simulink model "Quadcopter"  (R2023b)
settings: Solver=VariableStepAuto  StartTime=0.0  StopTime=30  RelTol=1e-3
values from neighbouring files (symbols this model uses):
  Pobs1x = zeros(1, length(Ob1))    [UAVsAnimation.m]    (also in UAVs_TwoObstacles.m)
  Pobs1y = zeros(1, length(Ob1))    [UAVsAnimation.m]    (also in UAVs_TwoObstacles.m)
  Pobs1z = zeros(1, length(Ob1))    [UAVsAnimation.m]    (also in UAVs_TwoObstacles.m)
  Pobs2x = zeros(1, length(Ob2))    [UAVsAnimation.m]    (also in UAVs_TwoObstacles.m)
  Pobs2y = zeros(1, length(Ob2))    [UAVsAnimation.m]    (also in UAVs_TwoObstacles.m)
  Pobs2z = zeros(1, length(Ob2))    [UAVsAnimation.m]    (also in UAVs_TwoObstacles.m)
  X = x(:,1)    [UAVs_TwoObstacles.m]
  xd = cell2mat(Xd)    [UAVs_TwoObstacles.m]
  Y = x(:,2)    [UAVs_TwoObstacles.m]
  yd = cell2mat(Yd)    [UAVs_TwoObstacles.m]
  Z = x(:,3)    [UAVs_TwoObstacles.m]
  zd = cell2mat(Zd)    [UAVs_TwoObstacles.m]
libraries: sim3dlib x5, slpidlib x1
settings Model: Creator=The MathWorks, Inc.  LastModifiedBy=galil
settings OptimizationCC: ReuseModelBlockBuffer=off

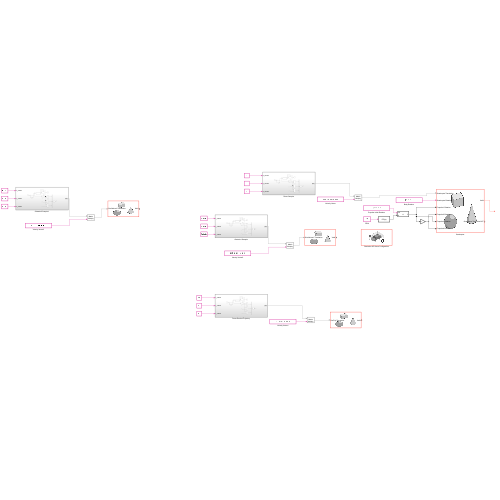
[thumbnail: Simulink's stored preview of the top-level diagram]
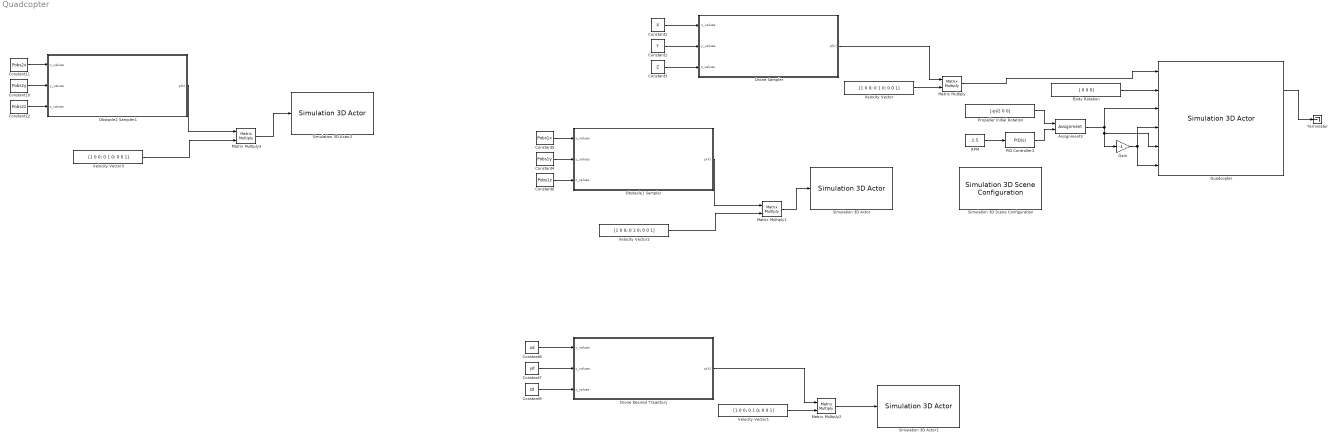
== system Quadcopter ==
  Assignment3 : Assignment  DiagnosticForDimensions=Warning  IndexOptions=Index vector (dialog)  Indices=3  OutputSizes=1
  Body Rotation : Constant  Value=[ 0 0 0]  VectorParams1D=off
  Constant1 : Constant  Value=Y
  Constant10 : Constant  Value=Pobs2y
  Constant11 : Constant  Value=Pobs2x
  Constant12 : Constant  Value=Pobs2z
  Constant2 : Constant  Value=X
  Constant3 : Constant  Value=Z
  Constant4 : Constant  Value=Pobs1y
  Constant5 : Constant  Value=Pobs1x
  Constant6 : Constant  Value=Pobs1z
  Constant7 : Constant  Value=yd
  Constant8 : Constant  Value=xd
  Constant9 : Constant  Value=zd
  Drone Desired Trajectory : Subsystem
  Drone Sampler : Subsystem
  Gain : Gain  Gain=-1
  Matrix Multiply{,1..3} (4 alike) : Product  Multiplication=Matrix(*)
  Obstacle1 Sampler : Subsystem
  Obstacle2 Sampler1 : Subsystem
  PID Controller3 : slpidlib/PID Controller  Controller=PID  Form=Parallel  TimeDomain=Continuous-time  UseExternalTs=off  SampleTime=-1  IntegratorMethod=Forward Euler  FilterMethod=Forward Euler  ControllerParametersSource=internal  P=0  I=1  UseKiTs=off  D=0  N=100  UseFilter=on  TunerSelectOption=Transfer Function Based (PID Tuner App)  InitialConditionSource=internal  InitialConditionForIntegrator=0  InitialConditionForFilter=0  DifferentiatorICPrevScaledInput=0  ExternalReset=none  TrackingMode=off  Kt=1  LimitOutput=off  SatLimitsSource=internal  UpperSaturationLimit=inf  LowerSaturationLimit=-inf  LinearizeAsGain=on  AntiWindupMode=none  Kb=1  LimitIntegrator=off  UpperIntegratorSaturationLimit=inf  LowerIntegratorSaturationLimit=-inf  POutMin=[]  POutMax=[]  IOutMin=[]  IOutMax=[]  DOutMin=[]  DOutMax=[]  NOutMin=[]  NOutMax=[]  SumOutMin=[]  SumOutMax=[]  SaturationOutMin=[]  SaturationOutMax=[]  PParamMin=[]  PParamMax=[]  IParamMin=[]  IParamMax=[]  DParamMin=[]  DParamMax=[]  NParamMin=[]  NParamMax=[]  KbParamMin=[]  KbParamMax=[]  KtParamMin=[]  KtParamMax=[]  KbOutMin=[]  KbOutMax=[]  KtOutMin=[]  KtOutMax=[]  IntegratorOutMin=[]  IntegratorOutMax=[]  FilterOutMin=[]  FilterOutMax=[]  SumI1OutMin=[]  SumI1OutMax=[]  SumI2OutMin=[]  SumI2OutMax=[]  SumI3OutMin=[]  SumI3OutMax=[]  SumI4OutMin=[]  SumI4OutMax=[]  SumDOutMin=[]  SumDOutMax=[]  DifferentiatorOutMin=[]  DifferentiatorOutMax=[]  FilterDiffOutCoefMin=[]  FilterDiffOutCoefMax=[]  ReciprocalOutMin=[]  ReciprocalOutMax=[]  SumDenOutMin=[]  SumDenOutMax=[]  SumNumOutMin=[]  SumNumOutMax=[]  DivideOutMin=[]  DivideOutMax=[]  UdiffTsProdOutMin=[]  UdiffTsProdOutMax=[]  NTsProdOutMin=[]  NTsProdOutMax=[]  UintegralTsProdOutMin=[]  UintegralTsProdOutMax=[]  UngainTsProdOutMin=[]  UngainTsProdOutMax=[]  ClampingZeroOutDataTypeStr=Inherit: Inherit via back propagation  ClampingZeroOutMin=[]  ClampingZeroOutMax=[]  FilterDenConstantOutDataTypeStr=Inherit: Inherit via back propagation  FilterDenConstantOutMin=[]  FilterDenConstantOutMax=[]  PCopyOutDataTypeStr=Inherit: Inherit via back propagation  PCopyOutMin=[]  PCopyOutMax=[]  NCopyOutDataTypeStr=Inherit: Inherit via back propagation  NCopyOutMin=[]  NCopyOutMax=[]  IntegratorContinuousStateAttributes=''  IntegratorStateMustResolveToSignalObject=off  IntegratorRTWStateStorageClass=Auto  FilterContinuousStateAttributes=''  FilterStateMustResolveToSignalObject=off  FilterRTWStateStorageClass=Auto  ParallelPVariant=InternalParameters  IdealPVariant=Disabled  IVariant=InternalParameters  DVariant=InternalParameters  IntegratorVariant=Continuous  SatVariant=Disabled  AWVariant=Passthrough  PCopyVariant=Disabled  TRVariant=Disabled  FdbkBlocksVariant=Forward  IdealPFdbkVariant=Disabled  SatFdbkVariant=Disabled  DerivativeFilterVariant=ContFilter  NVariant=InternalParameters  NCopyVariant=Disabled  FilterICVariant=InternalICsFilter  IntegratorICVariant=InternalICs  ExternalResetVariant=Disabled  TRSumVariant=Passthrough  SumFdbkVariant=Disabled  SumVariant=Sum_PID  TsampFilterVariant=InternalTs  TsampNgainVariant=Passthrough  TsampIntegralVariant=Disabled_SignalSpec  ExternalSaturationOutDataTypeStr=Inherit: Same as second input
  Propeller Initial Rotation : Constant  Value=[-pi/2 0 0]  VectorParams1D=off
  Quadcopter : sim3dlib/Simulation 3D Actor  ActorName=Quadcopter  ParentName=Scene Origin  Operation=Create at setup  InitScriptText=|  SampleTime=-1  Translation=single([-3.5 0 1.7])  Rotation=single([0 0 0])  Scale=single([1 1 1])  InputsText=|  OutputsText=Quadcopter.Translation  aMode=5  ActorTag=Quadcopter  ActorType=Sim3dActor  ID=C
      InitScriptText=|
      | fileName = "QuadCopter_Body.stl";
      | Body = sim3d.Actor('ActorName', 'Body', ...
      |     'Mobility', sim3d.utils.MobilityTypes.Movable, ...
      |     'ActorClassId', sim3d.utils.SemanticType.Vehicle);
      | World.add(Body, Actor);
      | Body.load(fileName, [1 1 1]/100);
      | Body.Rotation = [-pi/2 0 0 ];
      | Body.Color = [0, 0, 1];
      | Translation = [0.425 0.425 0.15;
      |     -0.425 0.425 0.15;
      |     0.425 -0.425 0.15;
      |     -0.425 -0.425 0.15];
      | propellerFileName = "QuadCopter_Propeller.stl";
      | for propellerIndex = 1:4
      | actorName = sprintf('Propeller%d', propellerIndex);
      | Propeller = sim3d.Actor('ActorName',actorName, ...
      |     'Mobility', sim3d.utils.MobilityTypes.Movable, ...
      |     'ActorClassId', sim3d.utils.SemanticType.Vehicle);
      | World.add(Propeller, Actor);
      | Propeller.load(propellerFileName, [1 1 1]/100);
      | Propeller.Color = [1, 0, 0];
      | Propeller.Translation = Translation(propellerIndex, :);
      | Propeller.Rotation = [-pi/2 0 0 ];
      | Actor.save("quadcopter.mat")
      | end
      InputsText=|
      | Quadcopter.Translation
      | Quadcopter.Rotation   
      | Propeller1.Rotation   
      | Propeller2.Rotation   
      | Propeller3.Rotation   
      | Propeller4.Rotation
      settings: LibrarySourceBlock=sl3dlib/Simulation 3D/Simulation 3D Actor
  RPM : Constant  Value=2.5
  Simulation 3D Actor : sim3dlib/Simulation 3D Actor  ActorName=Sim3dActor1  ParentName=Scene Origin  Operation=Create at setup  InitScriptText=|  SampleTime=-1  Translation=single([0 0 0])  Rotation=single([0 0 0])  Scale=single([1 1 1])  InputsText=Sim3dActor1.Translation  aMode=5  ActorTag=Sim3dActor1  ActorType=Sim3dActor  ID=1
      | Sim3dActor1 = sim3d.Actor('ActorName','Sim3dActor1', ...
      |     'Mobility', sim3d.utils.MobilityTypes.Movable, ...
      |     'ActorClassId', sim3d.utils.SemanticType.Vehicle);
      | createShape(Sim3dActor1,'sphere',[2 2 2]);
      | Sim3dActor1.Color = [1 1 1];
      | World.add(Sim3dActor1, Actor);
      settings: LibrarySourceBlock=sl3dlib/Simulation 3D/Simulation 3D Actor
  Simulation 3D Actor1 : sim3dlib/Simulation 3D Actor  ActorName=DesTraj  ParentName=Scene Origin  Operation=Create at setup  InitScriptText=|  SampleTime=-1  Translation=single([0 0 0])  Rotation=single([0 0 0])  Scale=single([1 1 1])  InputsText=DesTraj.Translation  aMode=5  ActorTag=DesTraj  ActorType=Sim3dActor  ID=C
      | fileName = "QuadCopter_Body.stl";
      | BodyDes = sim3d.Actor('ActorName', 'Body', ...
      |     'Mobility', sim3d.utils.MobilityTypes.Movable, ...
      |     'ActorClassId', sim3d.utils.SemanticType.Vehicle);
      | World.add(BodyDes, Actor);
      | BodyDes.load(fileName, [1 1 1]/100);
      | BodyDes.Rotation = [-pi/2 0 0 ];
      | BodyDes.Color = [0, 1, 0];
      | BodyDes.Transparency = 0.7;
      | Translation = [0.425 0.425 0.15;
      |     -0.425 0.425 0.15;
      |     0.425 -0.425 0.15;
      |     -0.425 -0.425 0.15];
      | propellerFileName = "QuadCopter_Propeller.stl";
      | for propellerIndex = 1:4
      | actorName = sprintf('Propeller%d', propellerIndex);
      | PropellerDes = sim3d.Actor('ActorName',actorName, ...
      |     'Mobility', sim3d.utils.MobilityTypes.Movable, ...
      |     'ActorClassId', sim3d.utils.SemanticType.Vehicle);
      | World.add(PropellerDes, Actor);
      | PropellerDes.load(propellerFileName, [1 1 1]/100);
      | PropellerDes.Color = [1, 0, 0];
      | PropellerDes.Translation = Translation(propellerIndex, :);
      | PropellerDes.Rotation = [-pi/2 0 0 ];
      | end
      settings: LibrarySourceBlock=sl3dlib/Simulation 3D/Simulation 3D Actor
  Simulation 3D Actor2 : sim3dlib/Simulation 3D Actor  ActorName=Sim3dActor2  ParentName=Scene Origin  Operation=Create at setup  InitScriptText=|  SampleTime=-1  Translation=single([0 0 0])  Rotation=single([0 0 0])  Scale=single([1 1 1])  InputsText=Sim3dActor2.Translation  aMode=5  ActorTag=Sim3dActor2  ActorType=Sim3dActor  ID=2
      | Sim3dActor2 = sim3d.Actor('ActorName','Sim3dActor2', ...
      |     'Mobility', sim3d.utils.MobilityTypes.Movable, ...
      |     'ActorClassId', sim3d.utils.SemanticType.Vehicle);
      | createShape(Sim3dActor2,'sphere',[2 2 2]);
      | Sim3dActor2.Color = [1 1 1];
      | World.add(Sim3dActor2, Actor);
      settings: LibrarySourceBlock=sl3dlib/Simulation 3D/Simulation 3D Actor
  Simulation 3D Scene Configuration : sim3dlib/Simulation 3D Scene Configuration  Priority=0  ProjectFormat=Default Scenes  SceneDesc=Empty scene  ProjectName=D:\Matlab\toolbox\shared\sim3d_projects\automotive_project_windows\UE\WindowsNoEditor\VehicleSimulation.exe  ScenePath=/Game/Maps/HwStrght  EnableOpenDRIVE=off  vehTagList={'Custom';'Quadcopter';'Scene Origin';'Sim3dActor1'}  vehTag=Custom  FreeCameraInitialTranslation=[0, -5, 20]  FreeCameraDefaultInitialTranslation=[-6, 0, 2]  FreeCameraInitialRotation=[0, 0, 90]  FreeCameraDefaultInitialRotation=[0, -15, 0]  OpVisEn=off  Ts=.02  EnableWindow=on  EnableRemoteAccess=off  EnableWeather=off  SunAltitude=40.0  SunAzimuth=90  clouds=10  wind=1  fog=0  rain=0  EnableGeospatial=off  OriginHeight=200  OriginLatitude=40.744652  OriginLongitude=-73.988864  MapStyle=Aerial  AdditionalAssetIDs=[]  UseAdvancedSunSky=off  SolarTime=11  TimeZone=-5  Day=21  Month=9  Year=2022  UseDaylightSavingTime=on  DSTStartDay=10  DSTStartMonth=3  DSTEndDay=3  DSTEndMonth=11  DSTSwitchHour=2  sensorTag=MainCamera2  sensorId=2  sensorName=MainCamera2  mountLoc=Origin  offsetFlag=off  tmountOffset=[0, 0, 0]  rmountOffset=[0, 0, 0]  HorizontalResolution=1280  VerticalResolution=720  HorizontalFOV=60  mountPoint=[0 0 0]  mountOrientation=[0 0 0]  aMode=5  ID=2  GeoTrigger=Inactive
      settings: LibrarySourceBlock=sl3dlib/Simulation 3D/Simulation 3D Scene Configuration
  Terminator : Terminator
  Velocity Vector{,1..3} (4 alike) : Constant  Value=[1 0 0; 0 1 0; 0 0 1]  VectorParams1D=off
  wires:
  RPM/1 -> PID Controller3/1
  PID Controller3/1 -> Assignment3/2
  Propeller Initial Rotation/1 -> Assignment3/1
  Assignment3/1 -> Quadcopter/3, Quadcopter/5, Gain/1
  Gain/1 -> Quadcopter/4, Quadcopter/6
  Quadcopter/1 -> Terminator/1
  Body Rotation/1 -> Quadcopter/2
  Constant2/1 -> Drone Sampler/1(x_values)
  Constant3/1 -> Drone Sampler/3(z_values)
  Constant1/1 -> Drone Sampler/2(y_values)
  Matrix Multiply/1 -> Quadcopter/1
  Drone Sampler/1(p(k)) -> Matrix Multiply/1
  Velocity Vector/1 -> Matrix Multiply/2
  Constant4/1 -> Obstacle1 Sampler/2(y_values)
  Constant5/1 -> Obstacle1 Sampler/1(x_values)
  Obstacle1 Sampler/1(p(k)) -> Matrix Multiply1/1
  Constant6/1 -> Obstacle1 Sampler/3(z_values)
  Velocity Vector2/1 -> Matrix Multiply1/2
  Matrix Multiply1/1 -> Simulation 3D Actor/1
  Constant7/1 -> Drone Desired Trajectory/2(y_values)
  Constant9/1 -> Drone Desired Trajectory/3(z_values)
  Constant8/1 -> Drone Desired Trajectory/1(x_values)
  Velocity Vector1/1 -> Matrix Multiply2/2
  Drone Desired Trajectory/1(p(k)) -> Matrix Multiply2/1
  Matrix Multiply2/1 -> Simulation 3D Actor1/1
  Constant10/1 -> Obstacle2 Sampler1/2(y_values)
  Obstacle2 Sampler1/1(p(k)) -> Matrix Multiply3/1
  Velocity Vector3/1 -> Matrix Multiply3/2
  Constant12/1 -> Obstacle2 Sampler1/3(z_values)
  Matrix Multiply3/1 -> Simulation 3D Actor2/1
  Constant11/1 -> Obstacle2 Sampler1/1(x_values)

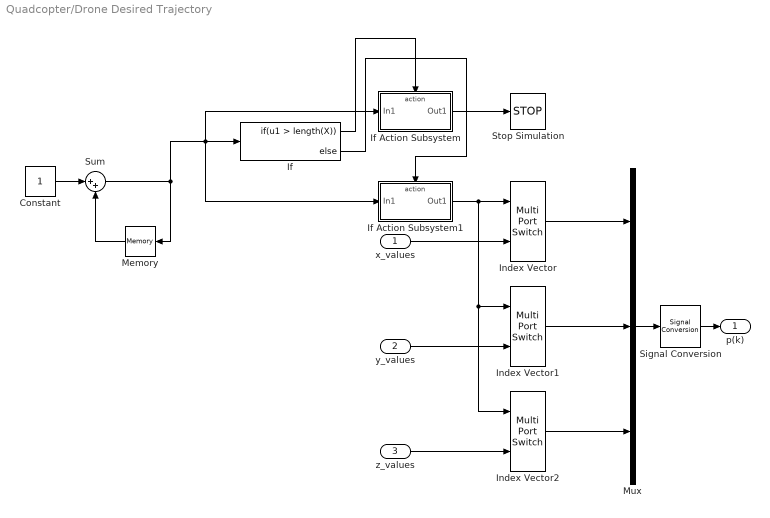
== system Quadcopter/Drone Desired Trajectory ==
  x_values : Inport
  y_values : Inport  Port=2
  z_values : Inport  Port=3
  Constant : Constant
  If : If  IfExpression=u1 > length(X)
  If Action Subsystem : Subsystem  TreatAsAtomicUnit=on
  If Action Subsystem1 : Subsystem  TreatAsAtomicUnit=on
  Index Vector : MultiPortSwitch  Inputs=1  SaturateOnIntegerOverflow=off  InputSameDT=off
  Index Vector1 : MultiPortSwitch  Inputs=1  SaturateOnIntegerOverflow=off  InputSameDT=off
  Index Vector2 : MultiPortSwitch  Inputs=1  SaturateOnIntegerOverflow=off  InputSameDT=off
  Memory : Memory
  Mux : Mux  Inputs=3
  Signal Conversion : SignalConversion  OverrideOpt=off
  Stop Simulation : Stop
  Sum : Sum  Inputs=|++
  p(k) : Outport
  wires:
  x_values/1 -> Index Vector/2
  If Action Subsystem/1(Out1) -> Stop Simulation/1
  If Action Subsystem1/1(Out1) -> Index Vector/1, Index Vector1/1, Index Vector2/1
  If/1 -> If Action Subsystem/Action
  Memory/1 -> Sum/2
  Sum/1 -> If Action Subsystem/1(In1), If/1, If Action Subsystem1/1(In1), Memory/1
  If/2 -> If Action Subsystem1/Action
  Constant/1 -> Sum/1
  y_values/1 -> Index Vector1/2
  z_values/1 -> Index Vector2/2
  Index Vector1/1 -> Mux/2
  Index Vector/1 -> Mux/1
  Index Vector2/1 -> Mux/3
  Mux/1 -> Signal Conversion/1
  Signal Conversion/1 -> p(k)/1

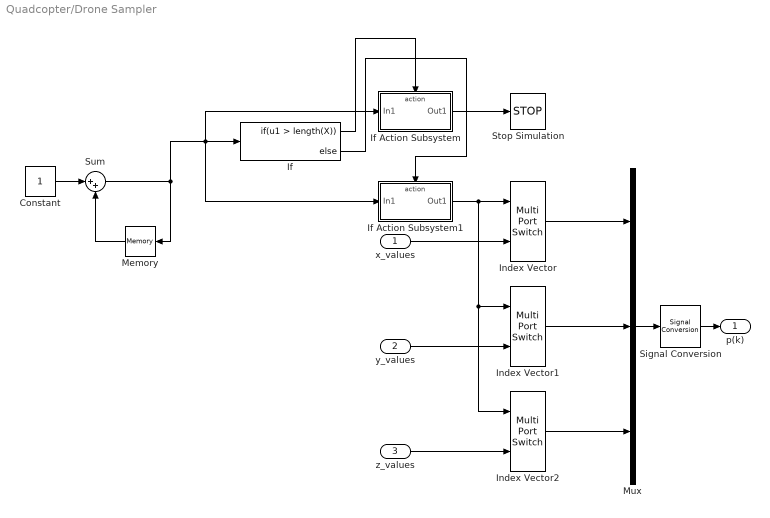
== system Quadcopter/Drone Sampler ==
  x_values : Inport
  y_values : Inport  Port=2
  z_values : Inport  Port=3
  Constant : Constant
  If : If  IfExpression=u1 > length(X)
  If Action Subsystem : Subsystem  TreatAsAtomicUnit=on
  If Action Subsystem1 : Subsystem  TreatAsAtomicUnit=on
  Index Vector : MultiPortSwitch  Inputs=1  SaturateOnIntegerOverflow=off  InputSameDT=off
  Index Vector1 : MultiPortSwitch  Inputs=1  SaturateOnIntegerOverflow=off  InputSameDT=off
  Index Vector2 : MultiPortSwitch  Inputs=1  SaturateOnIntegerOverflow=off  InputSameDT=off
  Memory : Memory
  Mux : Mux  Inputs=3
  Signal Conversion : SignalConversion  OverrideOpt=off
  Stop Simulation : Stop
  Sum : Sum  Inputs=|++
  p(k) : Outport
  wires:
  x_values/1 -> Index Vector/2
  If Action Subsystem/1(Out1) -> Stop Simulation/1
  If Action Subsystem1/1(Out1) -> Index Vector/1, Index Vector1/1, Index Vector2/1
  If/1 -> If Action Subsystem/Action
  Memory/1 -> Sum/2
  Sum/1 -> If Action Subsystem/1(In1), If/1, If Action Subsystem1/1(In1), Memory/1
  If/2 -> If Action Subsystem1/Action
  Constant/1 -> Sum/1
  y_values/1 -> Index Vector1/2
  z_values/1 -> Index Vector2/2
  Index Vector1/1 -> Mux/2
  Index Vector/1 -> Mux/1
  Index Vector2/1 -> Mux/3
  Mux/1 -> Signal Conversion/1
  Signal Conversion/1 -> p(k)/1

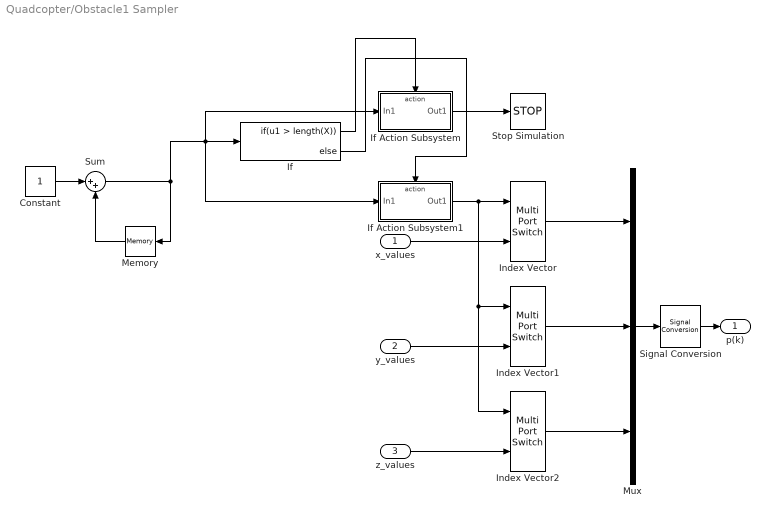
== system Quadcopter/Obstacle1 Sampler ==
  x_values : Inport
  y_values : Inport  Port=2
  z_values : Inport  Port=3
  Constant : Constant
  If : If  IfExpression=u1 > length(X)
  If Action Subsystem : Subsystem  TreatAsAtomicUnit=on
  If Action Subsystem1 : Subsystem  TreatAsAtomicUnit=on
  Index Vector : MultiPortSwitch  Inputs=1  SaturateOnIntegerOverflow=off  InputSameDT=off
  Index Vector1 : MultiPortSwitch  Inputs=1  SaturateOnIntegerOverflow=off  InputSameDT=off
  Index Vector2 : MultiPortSwitch  Inputs=1  SaturateOnIntegerOverflow=off  InputSameDT=off
  Memory : Memory
  Mux : Mux  Inputs=3
  Signal Conversion : SignalConversion  OverrideOpt=off
  Stop Simulation : Stop
  Sum : Sum  Inputs=|++
  p(k) : Outport
  wires:
  x_values/1 -> Index Vector/2
  If Action Subsystem/1(Out1) -> Stop Simulation/1
  If Action Subsystem1/1(Out1) -> Index Vector/1, Index Vector1/1, Index Vector2/1
  If/1 -> If Action Subsystem/Action
  Memory/1 -> Sum/2
  Sum/1 -> If Action Subsystem/1(In1), If/1, If Action Subsystem1/1(In1), Memory/1
  If/2 -> If Action Subsystem1/Action
  Constant/1 -> Sum/1
  y_values/1 -> Index Vector1/2
  z_values/1 -> Index Vector2/2
  Index Vector1/1 -> Mux/2
  Index Vector/1 -> Mux/1
  Index Vector2/1 -> Mux/3
  Mux/1 -> Signal Conversion/1
  Signal Conversion/1 -> p(k)/1

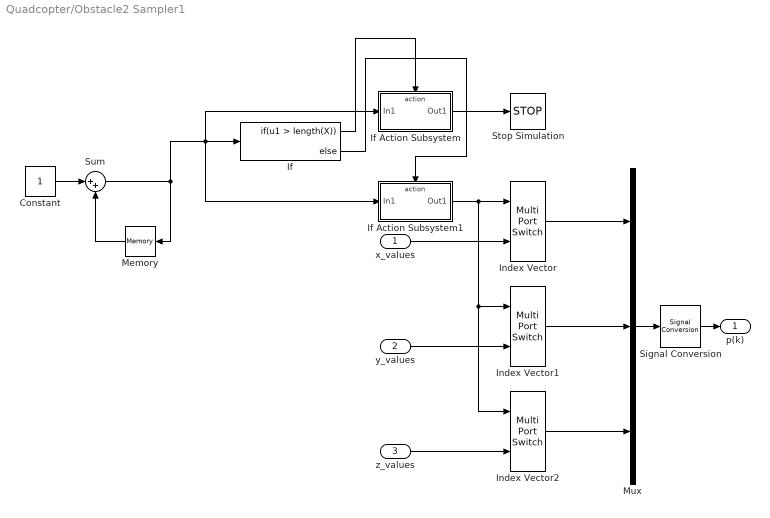
== system Quadcopter/Obstacle2 Sampler1 ==
  x_values : Inport
  y_values : Inport  Port=2
  z_values : Inport  Port=3
  Constant : Constant
  If : If  IfExpression=u1 > length(X)
  If Action Subsystem : Subsystem  TreatAsAtomicUnit=on
  If Action Subsystem1 : Subsystem  TreatAsAtomicUnit=on
  Index Vector : MultiPortSwitch  Inputs=1  SaturateOnIntegerOverflow=off  InputSameDT=off
  Index Vector1 : MultiPortSwitch  Inputs=1  SaturateOnIntegerOverflow=off  InputSameDT=off
  Index Vector2 : MultiPortSwitch  Inputs=1  SaturateOnIntegerOverflow=off  InputSameDT=off
  Memory : Memory
  Mux : Mux  Inputs=3
  Signal Conversion : SignalConversion  OverrideOpt=off
  Stop Simulation : Stop
  Sum : Sum  Inputs=|++
  p(k) : Outport
  wires:
  x_values/1 -> Index Vector/2
  If Action Subsystem/1(Out1) -> Stop Simulation/1
  If Action Subsystem1/1(Out1) -> Index Vector/1, Index Vector1/1, Index Vector2/1
  If/1 -> If Action Subsystem/Action
  Memory/1 -> Sum/2
  Sum/1 -> If Action Subsystem/1(In1), If/1, If Action Subsystem1/1(In1), Memory/1
  If/2 -> If Action Subsystem1/Action
  Constant/1 -> Sum/1
  y_values/1 -> Index Vector1/2
  z_values/1 -> Index Vector2/2
  Index Vector1/1 -> Mux/2
  Index Vector/1 -> Mux/1
  Index Vector2/1 -> Mux/3
  Mux/1 -> Signal Conversion/1
  Signal Conversion/1 -> p(k)/1

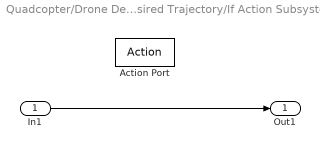
== system Quadcopter/Drone Desired Trajectory/If Action Subsystem ==
  In1 : Inport
  Action Port : ActionPort  ActionPortLabel=if(u1 > length(X))
  Out1 : Outport
  wires:
  In1/1 -> Out1/1

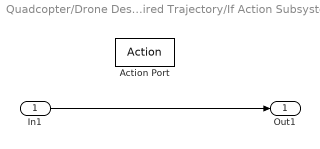
== system Quadcopter/Drone Desired Trajectory/If Action Subsystem1 ==
  In1 : Inport
  Action Port : ActionPort  ActionPortLabel=else
  Out1 : Outport
  wires:
  In1/1 -> Out1/1

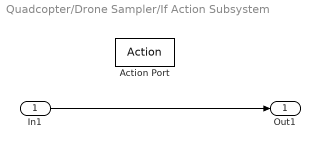
== system Quadcopter/Drone Sampler/If Action Subsystem ==
  In1 : Inport
  Action Port : ActionPort  ActionPortLabel=if(u1 > length(X))
  Out1 : Outport
  wires:
  In1/1 -> Out1/1

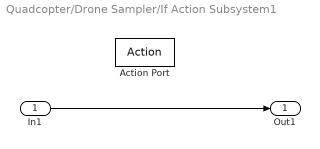
== system Quadcopter/Drone Sampler/If Action Subsystem1 ==
  In1 : Inport
  Action Port : ActionPort  ActionPortLabel=else
  Out1 : Outport
  wires:
  In1/1 -> Out1/1

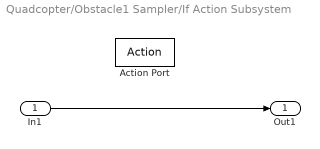
== system Quadcopter/Obstacle1 Sampler/If Action Subsystem ==
  In1 : Inport
  Action Port : ActionPort  ActionPortLabel=if(u1 > length(X))
  Out1 : Outport
  wires:
  In1/1 -> Out1/1

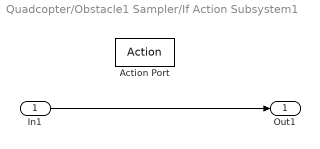
== system Quadcopter/Obstacle1 Sampler/If Action Subsystem1 ==
  In1 : Inport
  Action Port : ActionPort  ActionPortLabel=else
  Out1 : Outport
  wires:
  In1/1 -> Out1/1

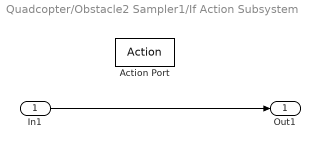
== system Quadcopter/Obstacle2 Sampler1/If Action Subsystem ==
  In1 : Inport
  Action Port : ActionPort  ActionPortLabel=if(u1 > length(X))
  Out1 : Outport
  wires:
  In1/1 -> Out1/1

== system Quadcopter/Obstacle2 Sampler1/If Action Subsystem1 ==
  In1 : Inport
  Action Port : ActionPort  ActionPortLabel=else
  Out1 : Outport
  wires:
  In1/1 -> Out1/1
